simulink model "Supervisory Control Development Simulink Model"  (R2024b)
settings: Solver=ode1  StartTime=0.0  StopTime=100.0  FixedStep=0.001  RelTol=1e-3
undefined symbols (not defined in the file): A, C_d, Crr, eta, g, m, max_veh, rho
libraries: slpidlib x1
settings Model: Creator=Ryan Sequeira  LastModifiedBy=Ryan Sequeira
settings SolverCC: DecoupledContinuousIntegration=on
settings DebuggingCC: ReadBeforeWriteMsg=DisableAll  WriteAfterWriteMsg=DisableAll  WriteAfterReadMsg=DisableAll  MultiTaskDSMMsg=none
settings ModelReferenceCC: UpdateModelReferenceTargets=IfOutOfDate
settings SFSimCC: SFSimEcho=off

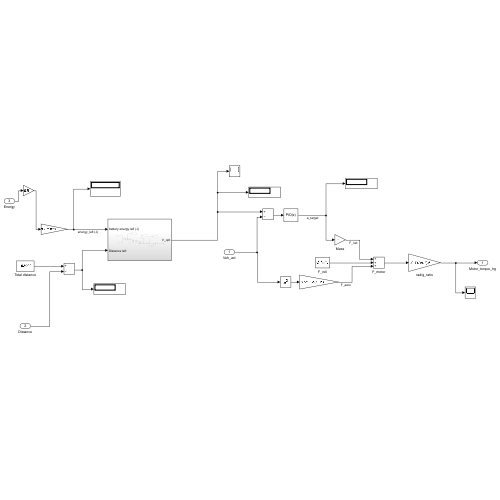
[thumbnail: Simulink's stored preview of the top-level diagram]
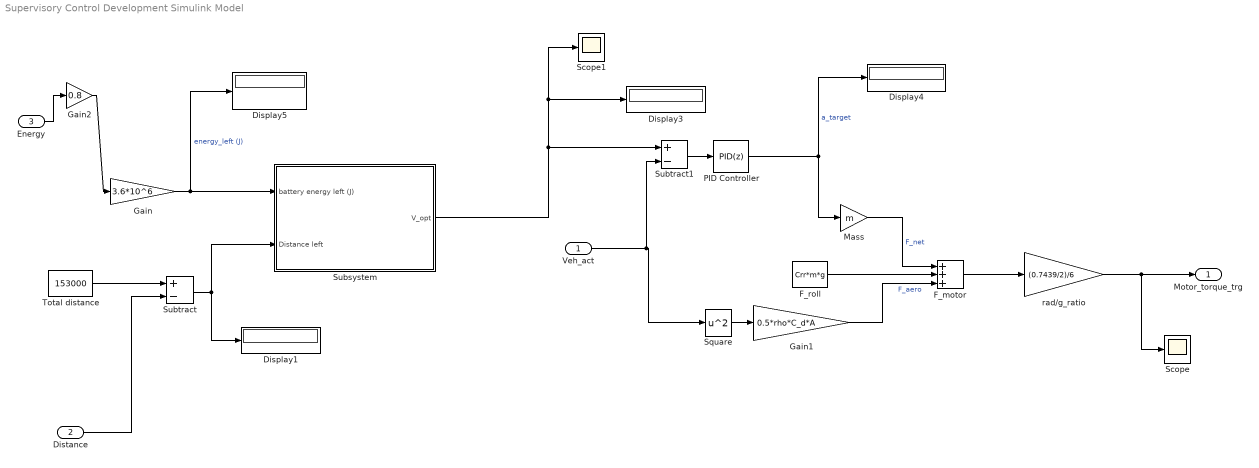
== system Supervisory Control Development Simulink Model ==
  Veh_act : Inport
  Distance : Inport  Port=2
  Energy : Inport  Port=3
  Display{1,3..5} (4 alike) : Display
  F_motor : Sum  Inputs=+++
  F_roll : Constant  Value=Crr*m*g
  Gain : Gain  Gain=3.6*10^6
  Gain1 : Gain  Gain=0.5*rho*C_d*A
  Gain2 : Gain  Gain=0.8
  Mass : Gain  Gain=m
  PID Controller : slpidlib/PID Controller  Controller=PID  Form=Parallel  TimeDomain=Discrete-time  UseExternalTs=off  SampleTime=-1  IntegratorMethod=Forward Euler  FilterMethod=Forward Euler  ControllerParametersSource=internal  P=0.4  I=0.000001  UseKiTs=off  D=0  UseExternalDerivativeSource=off  N=100  UseFilter=on  TunerSelectOption=Transfer Function Based (PID Tuner App)  InitialConditionSource=internal  InitialConditionForIntegrator=0  InitialConditionForFilter=0  DifferentiatorICPrevScaledInput=0  ExternalReset=none  TrackingMode=off  Kt=1  LimitOutput=off  SatLimitsSource=internal  UpperSaturationLimit=inf  LowerSaturationLimit=-inf  LinearizeAsGain=on  AntiWindupMode=none  Kb=1  LimitIntegrator=off  UpperIntegratorSaturationLimit=inf  LowerIntegratorSaturationLimit=-inf  POutMin=[]  POutMax=[]  IOutMin=[]  IOutMax=[]  DOutMin=[]  DOutMax=[]  NOutMin=[]  NOutMax=[]  SumOutMin=[]  SumOutMax=[]  SaturationOutMin=[]  SaturationOutMax=[]  PParamMin=[]  PParamMax=[]  IParamMin=[]  IParamMax=[]  DParamMin=[]  DParamMax=[]  NParamMin=[]  NParamMax=[]  KbParamMin=[]  KbParamMax=[]  KtParamMin=[]  KtParamMax=[]  KbOutMin=[]  KbOutMax=[]  KtOutMin=[]  KtOutMax=[]  IntegratorOutMin=[]  IntegratorOutMax=[]  FilterOutMin=[]  FilterOutMax=[]  SumI1OutMin=[]  SumI1OutMax=[]  SumI2OutMin=[]  SumI2OutMax=[]  SumI3OutMin=[]  SumI3OutMax=[]  SumI4OutMin=[]  SumI4OutMax=[]  SumDOutMin=[]  SumDOutMax=[]  DifferentiatorOutMin=[]  DifferentiatorOutMax=[]  FilterDiffOutCoefMin=[]  FilterDiffOutCoefMax=[]  ReciprocalOutMin=[]  ReciprocalOutMax=[]  SumDenOutMin=[]  SumDenOutMax=[]  SumNumOutMin=[]  SumNumOutMax=[]  DivideOutMin=[]  DivideOutMax=[]  UdiffTsProdOutMin=[]  UdiffTsProdOutMax=[]  NTsProdOutMin=[]  NTsProdOutMax=[]  UintegralTsProdOutMin=[]  UintegralTsProdOutMax=[]  UngainTsProdOutMin=[]  UngainTsProdOutMax=[]  ClampingZeroOutDataTypeStr=Inherit: Inherit via back propagation  ClampingZeroOutMin=[]  ClampingZeroOutMax=[]  FilterDenConstantOutDataTypeStr=Inherit: Inherit via back propagation  FilterDenConstantOutMin=[]  FilterDenConstantOutMax=[]  PCopyOutDataTypeStr=Inherit: Inherit via back propagation  PCopyOutMin=[]  PCopyOutMax=[]  NCopyOutDataTypeStr=Inherit: Inherit via back propagation  NCopyOutMin=[]  NCopyOutMax=[]  IntegratorContinuousStateAttributes=''  IntegratorStateMustResolveToSignalObject=off  IntegratorRTWStateStorageClass=Auto  FilterContinuousStateAttributes=''  FilterStateMustResolveToSignalObject=off  FilterRTWStateStorageClass=Auto  ParallelPVariant=InternalParameters  IdealPVariant=Disabled  IVariant=InternalParameters  DVariant=InternalParameters  IntegratorVariant=Discrete  SatVariant=Disabled  AWVariant=Passthrough  PCopyVariant=Disabled  TRVariant=Disabled  FdbkBlocksVariant=Forward  IdealPFdbkVariant=Disabled  SatFdbkVariant=Disabled  DerivativeFilterVariant=ForwardEulerFilter  NVariant=InternalParameters  NCopyVariant=Disabled  FilterICVariant=InternalICsFilter  IntegratorICVariant=InternalICs  ExternalResetVariant=Disabled  TRSumVariant=Passthrough  SumFdbkVariant=Disabled  SumVariant=Sum_PID  TsampFilterVariant=InternalTs  TsampNgainVariant=Passthrough  TsampIntegralVariant=Disabled_SignalSpec  ExternalSaturationOutDataTypeStr=Inherit: Same as second input  DerivativeSourceVariant=ErrorSignal  PreIntVariant=InternalPreInt
  Scope : Scope
  Scope1 : Scope
  Square : Math  Operator=square
  Subsystem : Subsystem
  Subtract : Sum  Inputs=+-
  Subtract1 : Sum  Inputs=+-
  Total distance : Constant  Value=153000
  rad/g_ratio : Gain  Gain=(0.7439/2)/6
  Motor_torque_trg : Outport
  wires:
  Subtract/1 -> Subsystem/2(Distance left), Display1/1
  Gain/1 -> Display5/1, Subsystem/1(battery energy left (J))  "energy_left (J)"
  Total distance/1 -> Subtract/1
  PID Controller/1 -> Mass/1, Display4/1  "a_target"
  Subsystem/1(V_opt) -> Subtract1/1, Display3/1, Scope1/1
  Subtract1/1 -> PID Controller/1
  Square/1 -> Gain1/1
  F_roll/1 -> F_motor/2
  Mass/1 -> F_motor/1  "F_net"
  Gain1/1 -> F_motor/3  "F_aero"
  F_motor/1 -> rad/g_ratio/1
  Veh_act/1 -> Subtract1/2, Square/1
  Distance/1 -> Subtract/2
  Gain2/1 -> Gain/1
  Energy/1 -> Gain2/1
  rad/g_ratio/1 -> Scope/1, Motor_torque_trg/1

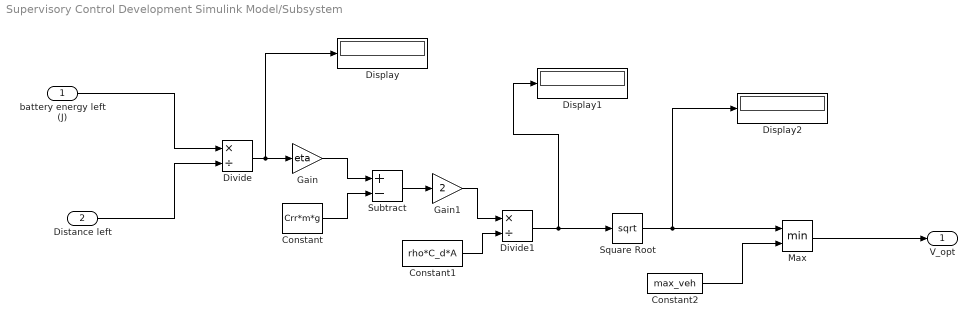
== system Supervisory Control Development Simulink Model/Subsystem ==
  battery energy left (J) : Inport
  Distance left : Inport  Port=2
  Constant : Constant  Value=Crr*m*g
  Constant1 : Constant  Value=rho*C_d*A
  Constant2 : Constant  Value=max_veh
  Display : Display
  Display1 : Display
  Display2 : Display
  Divide : Product  Inputs=*/
  Divide1 : Product  Inputs=*/
  Gain : Gain  Gain=eta
  Gain1 : Gain  Gain=2
  Max : MinMax  Inputs=2
  Square Root : Sqrt
  Subtract : Sum  Inputs=+-
  V_opt : Outport
  wires:
  battery energy left (J)/1 -> Divide/1
  Distance left/1 -> Divide/2
  Gain/1 -> Subtract/1
  Divide/1 -> Display/1, Gain/1
  Constant/1 -> Subtract/2
  Gain1/1 -> Divide1/1
  Subtract/1 -> Gain1/1
  Divide1/1 -> Square Root/1, Display1/1
  Constant1/1 -> Divide1/2
  Constant2/1 -> Max/2
  Square Root/1 -> Display2/1, Max/1
  Max/1 -> V_opt/1
